simulink model "lab2_model_challenge"  (R2024b)
settings: Solver=FixedStepAuto  StartTime=0.0  StopTime=sIn.simulation_time  FixedStep=sIn.step_size
undefined symbols (not defined in the file or in its folder): DiscIntNeverNeededParam, drv, feedback, gbox, mld, mot, obs, rads2rpm, rpm2rads, sens, sIn
libraries: simulink_extras x1
settings Model: Creator=bmm1  LastModifiedBy=Nihal
settings RTWCC: GPUComputeCapability=3.5

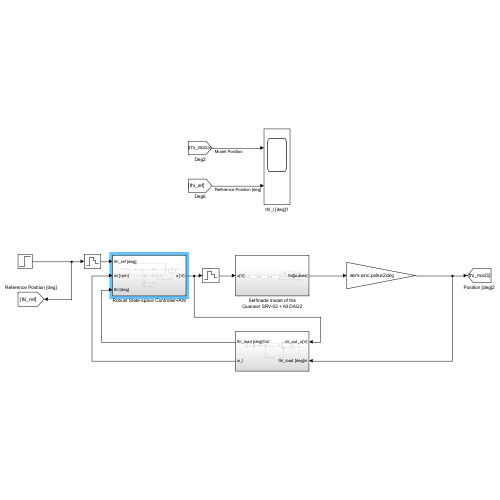
[thumbnail: Simulink's stored preview of the top-level diagram]
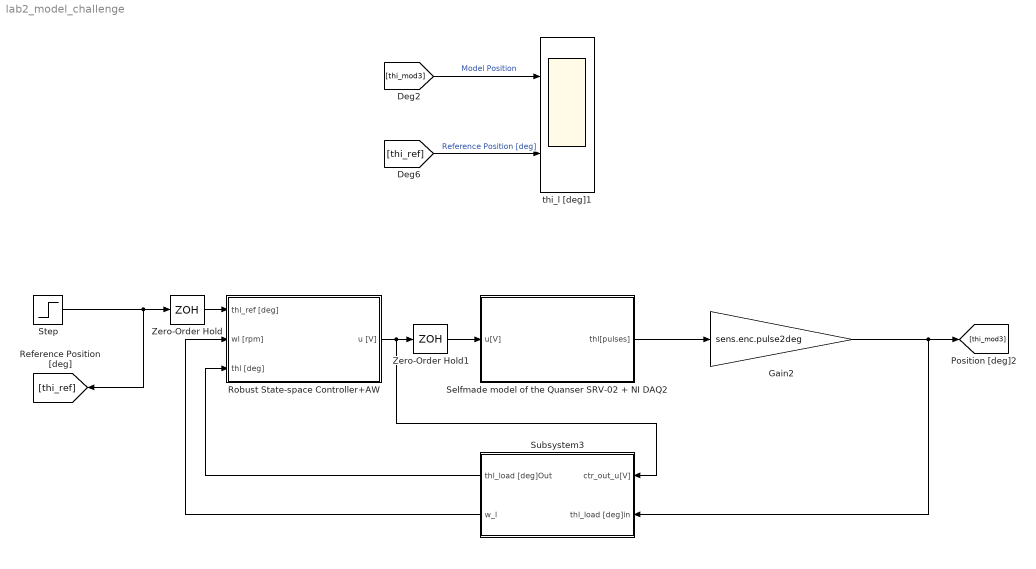
== system lab2_model_challenge ==
  Gain2 : Gain  Gain=sens.enc.pulse2deg
  Robust State-space Controller+AW : Subsystem
  Selfmade model of the Quanser SRV-02 + NI DAQ2 : Subsystem
  Step : Step  Time=0  After=60  SampleTime=0
  Subsystem3 : Subsystem
  Zero-Order Hold : ZeroOrderHold  SampleTime=sIn.T_s
  Zero-Order Hold1 : ZeroOrderHold  SampleTime=sIn.T_s
  thi_l [deg]1 : Scope  NumInputPorts=2
  wires:
  Selfmade model of the Quanser SRV-02 + NI DAQ2/1(thl[pulses]) -> Gain2/1
  Subsystem3/2(w_l) -> Robust State-space Controller+AW/2(wl [rpm])
  Gain2/1 -> [thi_mod3], Subsystem3/2(thl_load [deg]in)
  Subsystem3/1(thl_load [deg]Out) -> Robust State-space Controller+AW/3(thl [deg])
  Robust State-space Controller+AW/1(u [V]) -> Zero-Order Hold1/1, Subsystem3/1(ctr_out_u[V])
  Step/1 -> Zero-Order Hold/1, [thi_ref]
  Zero-Order Hold/1 -> Robust State-space Controller+AW/1(thl_ref [deg])
  Zero-Order Hold1/1 -> Selfmade model of the Quanser SRV-02 + NI DAQ2/1(u[V])
  [thi_ref] -> thi_l [deg]1/2  "Reference Position [deg]"
  [thi_mod3] -> thi_l [deg]1/1  "Model Position"

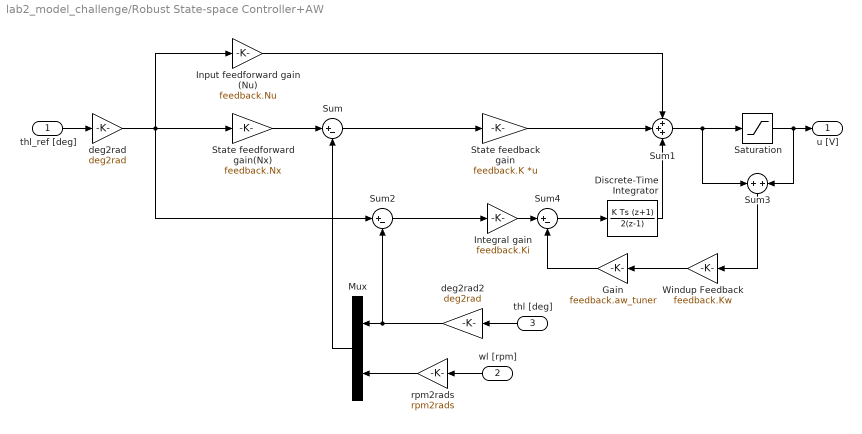
== system lab2_model_challenge/Robust State-space Controller+AW ==
  thl_ref [deg] : Inport
  wl [rpm] : Inport  Port=2
  thl [deg] : Inport  Port=3
  Discrete-Time Integrator : DiscreteIntegrator  IntegratorMethod=Integration: Trapezoidal  SampleTime=sIn.T_s  ICPrevOutput=DiscIntNeverNeededParam  ICPrevScaledInput=DiscIntNeverNeededParam
  Gain : Gain  Gain=feedback.aw_tuner
  Input feedforward gain (Nu) : Gain  Gain=feedback.Nu
  Integral gain : Gain  Gain=feedback.Ki
  Mux : Mux  Inputs=2
  Saturation : Saturate  UpperLimit=10  LowerLimit=-10
  State feedback gain : Gain  Gain=feedback.K  Multiplication=Matrix(K*u)
  State feedforward gain(Nx) : Gain  Gain=feedback.Nx
  Sum : Sum  Inputs=|+-
  Sum1 : Sum  Inputs=+++
  Sum2 : Sum  Inputs=|+-
  Sum3 : Sum  Inputs=+|+
  Sum4 : Sum  Inputs=|+-
  Windup Feedback : Gain  Gain=feedback.Kw
  deg2rad : Gain  Gain=deg2rad
  deg2rad2 : Gain  Gain=deg2rad
  rpm2rads : Gain  Gain=rpm2rads
  u [V] : Outport
  wires:
  thl_ref [deg]/1 -> deg2rad/1
  State feedforward gain(Nx)/1 -> Sum/1
  Sum/1 -> State feedback gain/1
  State feedback gain/1 -> Sum1/2
  Input feedforward gain (Nu)/1 -> Sum1/1
  Sum1/1 -> Sum3/1, Saturation/1
  Saturation/1 -> Sum3/2, u [V]/1
  thl [deg]/1 -> deg2rad2/1
  wl [rpm]/1 -> rpm2rads/1
  rpm2rads/1 -> Mux/2
  Mux/1 -> Sum/2
  deg2rad/1 -> Sum2/1, Input feedforward gain (Nu)/1, State feedforward gain(Nx)/1
  Discrete-Time Integrator/1 -> Sum1/3
  Sum2/1 -> Integral gain/1
  deg2rad2/1 -> Sum2/2, Mux/1
  Sum4/1 -> Discrete-Time Integrator/1
  Integral gain/1 -> Sum4/1
  Windup Feedback/1 -> Gain/1
  Sum3/1 -> Windup Feedback/1
  Gain/1 -> Sum4/2

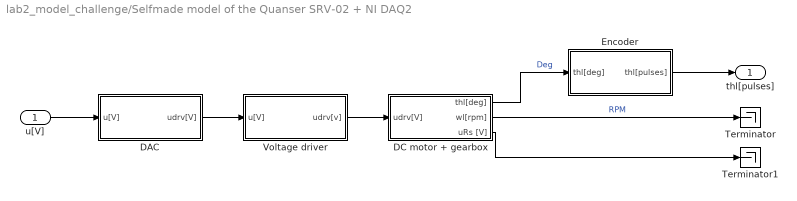
== system lab2_model_challenge/Selfmade model of the Quanser SRV-02 + NI DAQ2 ==
  u[V] : Inport
  DAC : Subsystem
  DC motor + gearbox : Subsystem
  Encoder : Subsystem
  Terminator : Terminator
  Terminator1 : Terminator
  Voltage driver : Subsystem
  thl[pulses] : Outport
  wires:
  DC motor + gearbox/1(thl[deg]) -> Encoder/1(thl[deg])  "Deg"
  u[V]/1 -> DAC/1(u[V])
  DC motor + gearbox/2(wl[rpm]) -> Terminator/1  "RPM"
  DAC/1(udrv[V]) -> Voltage driver/1(u[V])
  Voltage driver/1(udrv[v]) -> DC motor + gearbox/1(udrv[V])
  Encoder/1(thl[pulses]) -> thl[pulses]/1
  DC motor + gearbox/3(uRs [V]) -> Terminator1/1

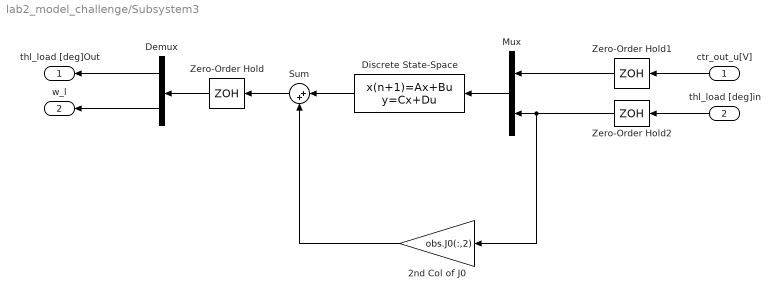
== system lab2_model_challenge/Subsystem3 ==
  ctr_out_u[V] : Inport
  thl_load [deg]in : Inport  Port=2
  2nd Col of J0 : Gain  Gain=obs.J0(:,2)
  Demux : Demux  Outputs=2
  Discrete State-Space : DiscreteStateSpace  A=obs.phi0  B=obs.gamma0  C=obs.H0  D=zeros(2,2)  SampleTime=sIn.T_s
  Mux : Mux  Inputs=2
  Sum : Sum  Inputs=|++
  Zero-Order Hold : ZeroOrderHold  SampleTime=sIn.T_s
  Zero-Order Hold1 : ZeroOrderHold  SampleTime=sIn.T_s
  Zero-Order Hold2 : ZeroOrderHold  SampleTime=sIn.T_s
  thl_load [deg]Out : Outport
  w_l : Outport  Port=2
  wires:
  Discrete State-Space/1 -> Sum/1
  Demux/2 -> w_l/1
  2nd Col of J0/1 -> Sum/2
  Demux/1 -> thl_load [deg]Out/1
  thl_load [deg]in/1 -> Zero-Order Hold2/1
  Mux/1 -> Discrete State-Space/1
  ctr_out_u[V]/1 -> Zero-Order Hold1/1
  Sum/1 -> Zero-Order Hold/1
  Zero-Order Hold1/1 -> Mux/1
  Zero-Order Hold2/1 -> 2nd Col of J0/1, Mux/2
  Zero-Order Hold/1 -> Demux/1

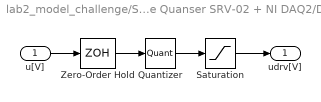
== system lab2_model_challenge/Selfmade model of the Quanser SRV-02 + NI DAQ2/DAC ==
  u[V] : Inport
  Quantizer : Quantizer  QuantizationInterval=daq.dac.q
  Saturation : Saturate  UpperLimit=10  LowerLimit=-10
  Zero-Order Hold : ZeroOrderHold  SampleTime=1e-3
  udrv[V] : Outport
  wires:
  Zero-Order Hold/1 -> Quantizer/1
  u[V]/1 -> Zero-Order Hold/1
  Quantizer/1 -> Saturation/1
  Saturation/1 -> udrv[V]/1

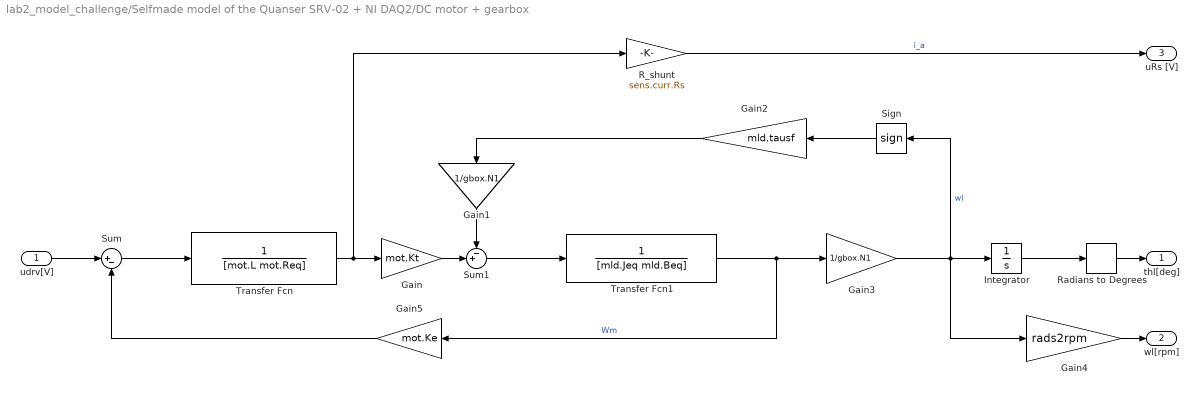
== system lab2_model_challenge/Selfmade model of the Quanser SRV-02 + NI DAQ2/DC motor + gearbox ==
  udrv[V] : Inport
  Gain : Gain  Gain=mot.Kt
  Gain1 : Gain  Gain=1/gbox.N1
  Gain2 : Gain  Gain=mld.tausf
  Gain3 : Gain  Gain=1/gbox.N1
  Gain4 : Gain  Gain=rads2rpm
  Gain5 : Gain  Gain=mot.Ke
  Integrator : Integrator
  R_shunt : Gain  Gain=sens.curr.Rs
  Radians to Degrees : simulink_extras/Transformations/Radians to Degrees
  Sign : Signum  ZeroCross=off
  Sum : Sum  Inputs=|+-
  Sum1 : Sum  Inputs=-+|
  Transfer Fcn : TransferFcn  Denominator=[mot.L mot.Req]
  Transfer Fcn1 : TransferFcn  Denominator=[mld.Jeq mld.Beq]
  thl[deg] : Outport
  wl[rpm] : Outport  Port=2
  uRs [V] : Outport  Port=3
  wires:
  udrv[V]/1 -> Sum/1
  Sum/1 -> Transfer Fcn/1
  Transfer Fcn/1 -> R_shunt/1, Gain/1
  Gain1/1 -> Sum1/1
  Gain2/1 -> Gain1/1
  Sign/1 -> Gain2/1
  Transfer Fcn1/1 -> Gain5/1, Gain3/1  "Wm"
  Gain3/1 -> Gain4/1, Sign/1, Integrator/1  "wl"
  Integrator/1 -> Radians to Degrees/1
  Radians to Degrees/1 -> thl[deg]/1
  Gain4/1 -> wl[rpm]/1
  Sum1/1 -> Transfer Fcn1/1
  Gain/1 -> Sum1/2
  Gain5/1 -> Sum/2
  R_shunt/1 -> uRs [V]/1  "i_a"

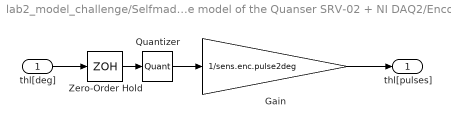
== system lab2_model_challenge/Selfmade model of the Quanser SRV-02 + NI DAQ2/Encoder ==
  thl[deg] : Inport
  Gain : Gain  Gain=1/sens.enc.pulse2deg
  Quantizer : Quantizer  QuantizationInterval=sens.enc.pulse2deg
  Zero-Order Hold : ZeroOrderHold  SampleTime=1e-3
  thl[pulses] : Outport
  wires:
  thl[deg]/1 -> Zero-Order Hold/1
  Gain/1 -> thl[pulses]/1
  Quantizer/1 -> Gain/1
  Zero-Order Hold/1 -> Quantizer/1

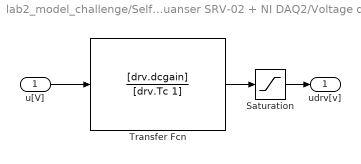
== system lab2_model_challenge/Selfmade model of the Quanser SRV-02 + NI DAQ2/Voltage driver ==
  u[V] : Inport
  Saturation : Saturate  UpperLimit=12  LowerLimit=-12
  Transfer Fcn : TransferFcn  Numerator=[drv.dcgain]  Denominator=[drv.Tc 1]
  udrv[v] : Outport
  wires:
  u[V]/1 -> Transfer Fcn/1
  Transfer Fcn/1 -> Saturation/1
  Saturation/1 -> udrv[v]/1
